simulink model "Example_Receiving_UDP_Video_In_Normal_Mode"  (R2016a)
settings: Solver=FixedStepAuto  StartTime=0.0  StopTime=inf  RelTol=1e-3
libraries: AR_Drone_Networking x1, visionsinks x1, dspnetwork x1, AR_Drone_Video_Processing x1
settings Model: Creator=sannem  LastModifiedBy=sannem

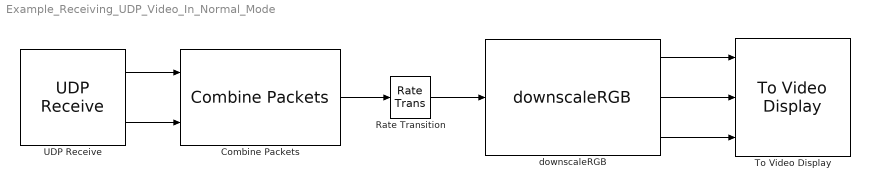
== system Example_Receiving_UDP_Video_In_Normal_Mode ==
  Combine Packets : AR_Drone_Networking/Combine Packets  fullPacketSize=73728
  Rate Transition : RateTransition  OutPortSampleTime=1/10
  To Video Display : visionsinks/To Video Display  windowSizeMode=True size (1:1)  openAtMdlStart=on  fullScreen=off  videoWindowX=0  videoWindowY=53  saveWindowSize=off  videoWindowWidth=1920  videoWindowHeight=1147  inputColorFormat=RGB  inputType=Obsolete  imagePorts=Separate color signals  OutputDevice=On-screen video monitor  dataOrg=Column-major  isWindowOpen=off
  UDP Receive : dspnetwork/UDP Receive  localURL='0.0.0.0'  localPort=24000  remoteURL='192.168.1.1'  remotePort=-1  recvBufferSize=73728  dims=15000  signalDatatype=uint8  isVarSize=off  showBlockingTime=off  blockingTime=0  sampletime=1/400
  "downscaleRGB " : AR_Drone_Video_Processing/downscaleRGB   width=1280/5  height=720/5  downScaleFactor=1
  wires:
  "downscaleRGB "/2 -> To Video Display/2
  "downscaleRGB "/1 -> To Video Display/1
  "downscaleRGB "/3 -> To Video Display/3
  Combine Packets/1 -> Rate Transition/1
  UDP Receive/1 -> Combine Packets/1
  Rate Transition/1 -> "downscaleRGB "/1
  UDP Receive/2 -> Combine Packets/2
